simulink model "cpu1"  (R2022b)
settings: Solver=FixedStepDiscrete  StartTime=0.0  StopTime=Inf  RelTol=1e-3  EnableMultiTasking=on
model workspace (MAT data in the model file):
  x = 1
undefined symbols (not defined in the file): C28x, CPU1, CPU2, EALLOW, EDIS
libraries: c2837xDlib x11, dspstat3 x5, c280xlib x5, slpidlib x2, c2802xlib x2, svdutilitieslib x1, dspswit3 x1, idelinklib_common x1
(part 1 of 2)
settings Model: ExtModeTrigDuration=8  Creator=asus  LastModifiedBy=KH
settings SolverCC: AlgebraicLoopSolver=TrustRegion  AutoInsertRateTranBlk=on  InsertRTBMode=Always
settings OptimizationCC: DefaultUnderspecifiedDataType=single  EnhancedBackFolding=on  PassReuseOutputArgsAs=Individual arguments  MaxStackSize=1024  OptimizeBlockOrder=speed  DifferentSizesBufferReuse=on  OptimizationCustomize=off  DenormalBehavior=FlushToZero  EfficientTunableParamExpr=on
settings DebuggingCC: ParameterPrecisionLossMsg=none  ParameterTunabilityLossMsg=error  UnconnectedInputMsg=warning  UnconnectedOutputMsg=warning  UnconnectedLineMsg=warning  SFMachineParentedDataDiag=warning
settings HardwareCC: ProdBitPerChar=16  ProdBitPerInt=16  ProdBitPerPointer=32  ProdBitPerSizeT=32  ProdBitPerPtrDiffT=32  ProdLargestAtomicInteger=Integer  ProdLargestAtomicFloat=None  ProdWordSize=16  ProdLongLongMode=on  ProdHWDeviceType=Texas Instruments->C2000
settings ModelReferenceCC: EnableRefExpFcnMdlSchedulingChecks=on
settings SFSimCC: MATLABDynamicMemAlloc=off
settings RTWCC: Description=Embedded Coder  SystemTargetFile=ert.tlc  HardwareBoard=TI Delfino F28379D LaunchPad  TLCOptions=-aInlineSetEventsForThisBaseRateFcn=TLC_FALSE -aSuppressMultiTaskScheduler=TLC_FALSE -aRateBasedStepFcn=1  TemplateMakefile=ert_default_tmf  Toolchain=Texas Instruments Code Composer Studio (C2000)  DLArmComputeVersion=19.05
settings CodeAppCC: ForceParamTrailComments=on  IgnoreCustomStorageClasses=off  OperatorAnnotations=on  SimulinkDataObjDesc=on  SFDataObjDesc=on  InsertBlockDesc=on
settings ERTTargetCC: CodeReplacementLibrary=TI C28x  ExtModeTransport=3  ExtModeStaticAllocSize=10000

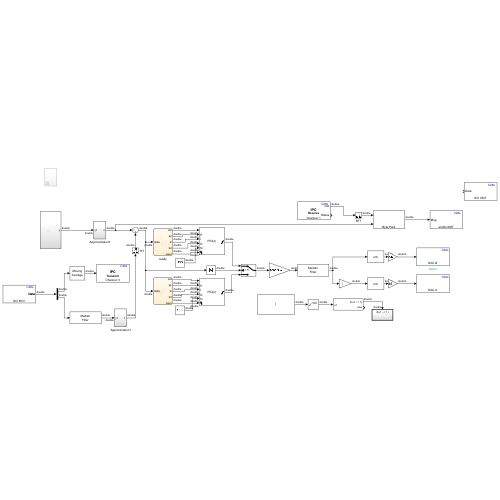
[thumbnail: Simulink's stored preview of the top-level diagram]
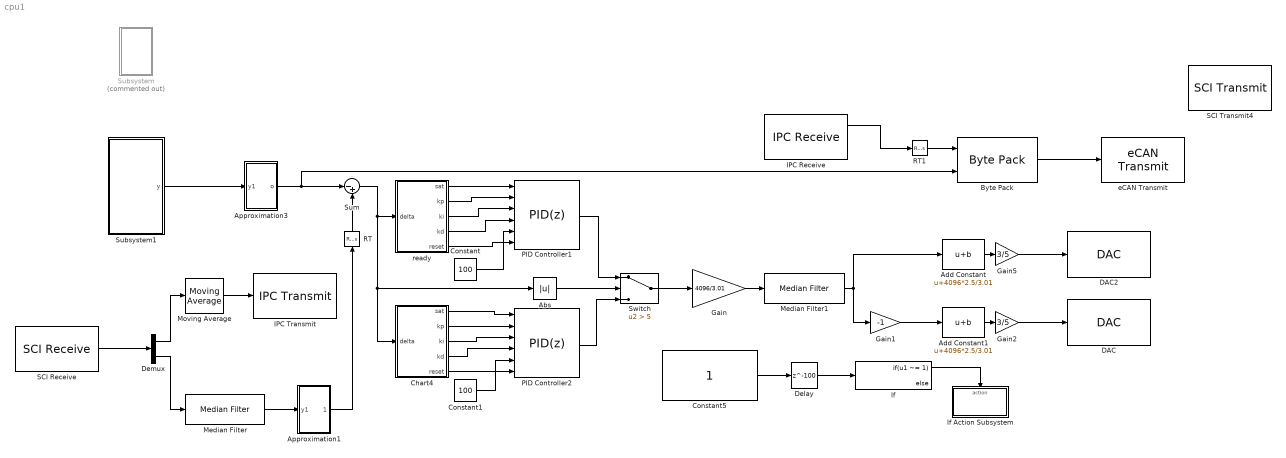
== system cpu1 ==
  " Approximation1" : Subsystem
  " Approximation3" : Subsystem
  Abs : Abs  SaturateOnIntegerOverflow=off
  Add Constant : Bias  Bias=4096*2.5/3.01  SaturateOnIntegerOverflow=off
  Add Constant1 : Bias  Bias=4096*2.5/3.01  SaturateOnIntegerOverflow=off
  Byte Pack : svdutilitieslib/Byte Pack  maskPackedDataType=uint16  datatypes={'single' 'single'}  byteAlign=4  blockPlatform=arduinoert
  Chart4 : Stateflow chart  TreatAsAtomicUnit=on
  Constant : Constant  Value=100
  Constant1 : Constant  Value=100
  Constant5 : Constant  OutDataTypeStr=Inherit: Inherit via back propagation
  DAC : c2837xDlib/DAC  channel=A  saturate=on
  DAC2 : c2837xDlib/DAC  channel=B  saturate=on
  Delay : Delay  DelayLength=100
  Demux : Demux  Outputs=2
  Gain : Gain  Gain=4096/3.01  OutDataTypeStr=single
  Gain1 : Gain  Gain=-1  OutDataTypeStr=single  SaturateOnIntegerOverflow=on
  Gain2 : Gain  Gain=3/5  OutDataTypeStr=single  SaturateOnIntegerOverflow=on
  Gain5 : Gain  Gain=3/5  OutDataTypeStr=single  SaturateOnIntegerOverflow=on
  IPC Receive : c2837xDlib/IPC Receive  blkParamProc=F2837x  SelectSource=C28x (CPU1/CPU2)  SelectChannel=1  DataType=single  DataLength=1  EnableBlocking=off  SampleTime=.001
  IPC Transmit : c2837xDlib/IPC Transmit  blkParamProc=F2837x  SelectDestination=C28x (CPU1/CPU2)  SelectChannel=0  EnableBlocking=off
  If : If  IfExpression=u1 ~= 1
  If Action Subsystem : Subsystem  TreatAsAtomicUnit=on
  Median Filter : dspstat3/Median Filter  WindowLength=3  SimulateUsing=Interpreted execution
  Median Filter1 : dspstat3/Median Filter  WindowLength=28  SimulateUsing=Interpreted execution
  Moving Average : dspstat3/Moving Average  Method=Sliding window  ForgettingFactorPort=off  SpecifyWindowLength=on  WindowLength=2  OverlapLength=1  AllowArbitraryInputLength=off  ForgettingFactor=0.9  SimulateUsing=Code generation
  PID Controller1 : slpidlib/PID Controller  Controller=PID  Form=Parallel  TimeDomain=Discrete-time  UseExternalTs=off  SampleTime=-1  IntegratorMethod=Forward Euler  FilterMethod=Forward Euler  ControllerParametersSource=external  P=0.0076  I=0.005  UseKiTs=off  D=0.00  N=100  UseFilter=on  TunerSelectOption=Transfer Function Based (PID Tuner App)  InitialConditionSource=internal  InitialConditionForIntegrator=0  InitialConditionForFilter=0  DifferentiatorICPrevScaledInput=0  ExternalReset=falling  TrackingMode=off  Kt=1  LimitOutput=on  SatLimitsSource=internal  UpperSaturationLimit=2.0  LowerSaturationLimit=-2.0  LinearizeAsGain=on  AntiWindupMode=clamping  Kb=1  LimitIntegrator=off  UpperIntegratorSaturationLimit=inf  LowerIntegratorSaturationLimit=-inf  PGainOutDataTypeStr=single  PProdOutDataTypeStr=single  POutMin=[]  POutMax=[]  IGainOutDataTypeStr=single  IProdOutDataTypeStr=single  IOutMin=[]  IOutMax=[]  DGainOutDataTypeStr=single  DProdOutDataTypeStr=single  DOutMin=[]  DOutMax=[]  NGainOutDataTypeStr=double  NProdOutDataTypeStr=double  NOutMin=[]  NOutMax=[]  SumOutDataTypeStr=single  SumOutMin=[]  SumOutMax=[]  SaturationOutDataTypeStr=single  SaturationOutMin=[]  SaturationOutMax=[]  PParamMin=[]  PParamMax=[]  IParamMin=[]  IParamMax=[]  DParamMin=[]  DParamMax=[]  NParamMin=[]  NParamMax=[]  KbParamMin=[]  KbParamMax=[]  KtParamMin=[]  KtParamMax=[]  KbOutMin=[]  KbOutMax=[]  KtOutMin=[]  KtOutMax=[]  IntegratorOutMin=[]  IntegratorOutMax=[]  FilterOutMin=[]  FilterOutMax=[]  SumI1OutMin=[]  SumI1OutMax=[]  SumI2OutMin=[]  SumI2OutMax=[]  SumI3OutMin=[]  SumI3OutMax=[]  SumI4OutMin=[]  SumI4OutMax=[]  SumDOutMin=[]  SumDOutMax=[]  DifferentiatorOutMin=[]  DifferentiatorOutMax=[]  FilterDiffOutCoefMin=[]  FilterDiffOutCoefMax=[]  ReciprocalOutMin=[]  ReciprocalOutMax=[]  SumDenOutMin=[]  SumDenOutMax=[]  SumNumOutMin=[]  SumNumOutMax=[]  DivideOutMin=[]  DivideOutMax=[]  UdiffTsProdOutMin=[]  UdiffTsProdOutMax=[]  NTsProdOutMin=[]  NTsProdOutMax=[]  UintegralTsProdOutMin=[]  UintegralTsProdOutMax=[]  UngainTsProdOutMin=[]  UngainTsProdOutMax=[]  ClampingZeroOutDataTypeStr=Inherit: Inherit via back propagation  ClampingZeroOutMin=[]  ClampingZeroOutMax=[]  FilterDenConstantOutDataTypeStr=Inherit: Inherit via back propagation  FilterDenConstantOutMin=[]  FilterDenConstantOutMax=[]  PCopyOutDataTypeStr=Inherit: Inherit via back propagation  PCopyOutMin=[]  PCopyOutMax=[]  NCopyOutDataTypeStr=Inherit: Inherit via back propagation  NCopyOutMin=[]  NCopyOutMax=[]  IntegratorContinuousStateAttributes=''  IntegratorStateMustResolveToSignalObject=off  IntegratorRTWStateStorageClass=Auto  FilterContinuousStateAttributes=''  FilterStateMustResolveToSignalObject=off  FilterRTWStateStorageClass=Auto  ParallelPVariant=ExternalParameters  IdealPVariant=Disabled  IVariant=ExternalParameters  DVariant=ExternalParameters  IntegratorVariant=Discrete  SatVariant=Enabled  AWVariant=DiscClampingParallel  PCopyVariant=Disabled  TRVariant=Disabled  FdbkBlocksVariant=Forward  IdealPFdbkVariant=Disabled  SatFdbkVariant=Disabled  DerivativeFilterVariant=ForwardEulerFilter  NVariant=ExternalParameters  NCopyVariant=Disabled  FilterICVariant=InternalICsFilter  IntegratorICVariant=InternalICs  ExternalResetVariant=ExternalReset  TRSumVariant=Passthrough  SumFdbkVariant=Disabled  SumVariant=Sum_PID  TsampFilterVariant=InternalTs  TsampNgainVariant=Passthrough  TsampIntegralVariant=Passthrough  ExternalSaturationOutDataTypeStr=Inherit: Same as second input
  PID Controller2 : slpidlib/PID Controller  Controller=PID  Form=Parallel  TimeDomain=Discrete-time  UseExternalTs=off  SampleTime=-1  IntegratorMethod=Forward Euler  FilterMethod=Forward Euler  ControllerParametersSource=external  P=0.0076  I=0.005  UseKiTs=off  D=0.00  N=100  UseFilter=on  TunerSelectOption=Transfer Function Based (PID Tuner App)  InitialConditionSource=internal  InitialConditionForIntegrator=0  InitialConditionForFilter=0  DifferentiatorICPrevScaledInput=0  ExternalReset=falling  TrackingMode=off  Kt=1  LimitOutput=on  SatLimitsSource=internal  UpperSaturationLimit=2.0  LowerSaturationLimit=-2.0  LinearizeAsGain=on  AntiWindupMode=none  Kb=1  LimitIntegrator=off  UpperIntegratorSaturationLimit=inf  LowerIntegratorSaturationLimit=-inf  PGainOutDataTypeStr=single  PProdOutDataTypeStr=single  POutMin=[]  POutMax=[]  IGainOutDataTypeStr=single  IProdOutDataTypeStr=single  IOutMin=[]  IOutMax=[]  DGainOutDataTypeStr=single  DProdOutDataTypeStr=single  DOutMin=[]  DOutMax=[]  NGainOutDataTypeStr=double  NProdOutDataTypeStr=double  NOutMin=[]  NOutMax=[]  SumOutDataTypeStr=single  SumOutMin=[]  SumOutMax=[]  SaturationOutDataTypeStr=single  SaturationOutMin=[]  SaturationOutMax=[]  PParamMin=[]  PParamMax=[]  IParamMin=[]  IParamMax=[]  DParamMin=[]  DParamMax=[]  NParamMin=[]  NParamMax=[]  KbParamMin=[]  KbParamMax=[]  KtParamMin=[]  KtParamMax=[]  KbOutMin=[]  KbOutMax=[]  KtOutMin=[]  KtOutMax=[]  IntegratorOutMin=[]  IntegratorOutMax=[]  FilterOutMin=[]  FilterOutMax=[]  SumI1OutMin=[]  SumI1OutMax=[]  SumI2OutMin=[]  SumI2OutMax=[]  SumI3OutMin=[]  SumI3OutMax=[]  SumI4OutMin=[]  SumI4OutMax=[]  SumDOutMin=[]  SumDOutMax=[]  DifferentiatorOutMin=[]  DifferentiatorOutMax=[]  FilterDiffOutCoefMin=[]  FilterDiffOutCoefMax=[]  ReciprocalOutMin=[]  ReciprocalOutMax=[]  SumDenOutMin=[]  SumDenOutMax=[]  SumNumOutMin=[]  SumNumOutMax=[]  DivideOutMin=[]  DivideOutMax=[]  UdiffTsProdOutMin=[]  UdiffTsProdOutMax=[]  NTsProdOutMin=[]  NTsProdOutMax=[]  UintegralTsProdOutMin=[]  UintegralTsProdOutMax=[]  UngainTsProdOutMin=[]  UngainTsProdOutMax=[]  ClampingZeroOutDataTypeStr=Inherit: Inherit via back propagation  ClampingZeroOutMin=[]  ClampingZeroOutMax=[]  FilterDenConstantOutDataTypeStr=Inherit: Inherit via back propagation  FilterDenConstantOutMin=[]  FilterDenConstantOutMax=[]  PCopyOutDataTypeStr=Inherit: Inherit via back propagation  PCopyOutMin=[]  PCopyOutMax=[]  NCopyOutDataTypeStr=Inherit: Inherit via back propagation  NCopyOutMin=[]  NCopyOutMax=[]  IntegratorContinuousStateAttributes=''  IntegratorStateMustResolveToSignalObject=off  IntegratorRTWStateStorageClass=Auto  FilterContinuousStateAttributes=''  FilterStateMustResolveToSignalObject=off  FilterRTWStateStorageClass=Auto  ParallelPVariant=ExternalParameters  IdealPVariant=Disabled  IVariant=ExternalParameters  DVariant=ExternalParameters  IntegratorVariant=Discrete  SatVariant=Enabled  AWVariant=Passthrough  PCopyVariant=Disabled  TRVariant=Disabled  FdbkBlocksVariant=Forward  IdealPFdbkVariant=Disabled  SatFdbkVariant=Disabled  DerivativeFilterVariant=ForwardEulerFilter  NVariant=ExternalParameters  NCopyVariant=Disabled  FilterICVariant=InternalICsFilter  IntegratorICVariant=InternalICs  ExternalResetVariant=ExternalReset  TRSumVariant=Passthrough  SumFdbkVariant=Disabled  SumVariant=Sum_PID  TsampFilterVariant=InternalTs  TsampNgainVariant=Passthrough  TsampIntegralVariant=Passthrough  ExternalSaturationOutDataTypeStr=Inherit: Same as second input
  RT : RateTransition  OutPortSampleTime=0.001
  RT1 : RateTransition  OutPortSampleTime=0.001
  SCI Receive : c280xlib/SCI Receive  sciModule=A  dataHead=''  headerCheckMaxCount=16  dataTail=''  dataType=single  dataLenOptions=Length via dialog  dataDim=2  maxDataLength=1  initValue=0  errOption=Output the last received value  errValue=0  sampleTime=0.1  blockingMode=on  timeOut=inf  outputStatus=off
  SCI Transmit4 : c280xlib/SCI Transmit  sciModule=A  dataHead=''  dataTail=''  blockingMode=on  outputStatus=off
  Subsystem : Subsystem  Commented=on
  Subsystem1 : Subsystem
  Sum : Sum  Inputs=|-+
  Switch : Switch  Criteria=u2 > Threshold  Threshold=5  SaturateOnIntegerOverflow=off  InputSameDT=off
  eCAN Transmit : c280xlib/eCAN Transmit  chipFamily=C280x  useModule=eCAN_A  mailboxNo=1  messageID=bin2dec('111000111')  messageType=Standard (11-bit identifier)  enableBlockingMode=off  postInterrupt=off  interruptLine=0
      settings: LibrarySourceBlock=c2837xDlib/eCAN Transmit
  ready : Stateflow chart  TreatAsAtomicUnit=on
  wires:
  If/1 -> If Action Subsystem/Action
  Delay/1 -> If/1
  Constant5/1 -> Delay/1
  Add Constant1/1 -> Gain2/1
  Add Constant/1 -> Gain5/1
  Gain1/1 -> Add Constant1/1
  Gain5/1 -> DAC2/1
  Gain2/1 -> DAC/1
  Constant/1 -> PID Controller1/5
  PID Controller1/1 -> Switch/1
  ready/2(kp) -> PID Controller1/2
  ready/3(ki) -> PID Controller1/3
  ready/4(kd) -> PID Controller1/4
  ready/1(sat) -> PID Controller1/1
  ready/5(reset) -> PID Controller1/6
  " Approximation1"/1(Out1) -> RT/1
  RT/1 -> Sum/2
  Subsystem1/1(y) -> " Approximation3"/1(y1)
  Median Filter/1 -> " Approximation1"/1(y1)
  Gain/1 -> Median Filter1/1
  " Approximation3"/1(o) -> Byte Pack/2, Sum/1
  Switch/1 -> Gain/1
  Chart4/5(reset) -> PID Controller2/6
  Chart4/1(sat) -> PID Controller2/1
  Chart4/3(ki) -> PID Controller2/3
  Constant1/1 -> PID Controller2/5
  Chart4/4(kd) -> PID Controller2/4
  Sum/1 -> Chart4/1(delta), Abs/1, ready/1(delta)
  Chart4/2(kp) -> PID Controller2/2
  PID Controller2/1 -> Switch/3
  Abs/1 -> Switch/2
  Median Filter1/1 -> Gain1/1, Add Constant/1
  Demux/1 -> Moving Average/1
  Moving Average/1 -> IPC Transmit/1
  IPC Receive/1 -> RT1/1
  RT1/1 -> Byte Pack/1
  SCI Receive/1 -> Demux/1
  Demux/2 -> Median Filter/1
  Byte Pack/1 -> eCAN Transmit/1

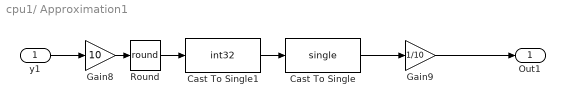
== system cpu1/ Approximation1 ==
  y1 : Inport
  Cast To Single : DataTypeConversion  OutDataTypeStr=single  SaturateOnIntegerOverflow=off  RndMeth=Floor
  Cast To Single1 : DataTypeConversion  OutDataTypeStr=int32  SaturateOnIntegerOverflow=off  RndMeth=Floor
  Gain8 : Gain  Gain=10
  Gain9 : Gain  Gain=1/10
  Round : Rounding  Operator=round
  Out1 : Outport
  wires:
  y1/1 -> Gain8/1
  Gain8/1 -> Round/1
  Round/1 -> Cast To Single1/1
  Cast To Single1/1 -> Cast To Single/1
  Cast To Single/1 -> Gain9/1
  Gain9/1 -> Out1/1

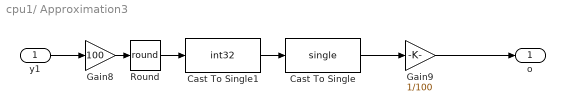
== system cpu1/ Approximation3 ==
  y1 : Inport
  Cast To Single : DataTypeConversion  OutDataTypeStr=single  SaturateOnIntegerOverflow=off  RndMeth=Floor
  Cast To Single1 : DataTypeConversion  OutDataTypeStr=int32  SaturateOnIntegerOverflow=off  RndMeth=Floor
  Gain8 : Gain  Gain=100
  Gain9 : Gain  Gain=1/100
  Round : Rounding  Operator=round
  o : Outport
  wires:
  Gain9/1 -> o/1
  Cast To Single/1 -> Gain9/1
  Cast To Single1/1 -> Cast To Single/1
  Round/1 -> Cast To Single1/1
  Gain8/1 -> Round/1
  y1/1 -> Gain8/1

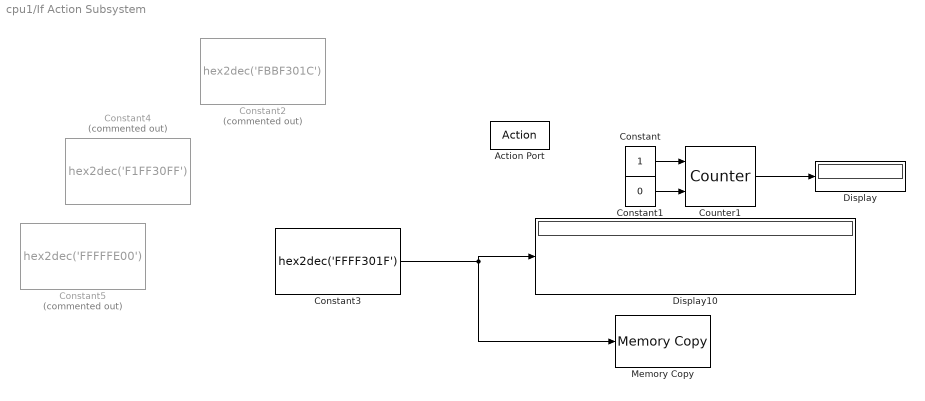
== system cpu1/If Action Subsystem ==
  Action Port : ActionPort  ActionPortLabel=if(u1 ~= 1)
  Constant : Constant
  Constant1 : Constant  Value=0
  Constant2 : Constant  Commented=on  Value=hex2dec('FBBF301C')  OutDataTypeStr=uint32
  Constant3 : Constant  Value=hex2dec('FFFF301F')  OutDataTypeStr=uint32
  Constant4 : Constant  Commented=on  Value=hex2dec('F1FF30FF')  OutDataTypeStr=uint32
  Constant5 : Constant  Commented=on  Value=hex2dec('FFFFFE00')  OutDataTypeStr=uint32
  Counter1 : dspswit3/Counter  Direction=Up  CountEvent=Rising edge  CounterSize=User defined  MaxCount=255  InitialCount=0  Output=Count  HitValue=32  ResetInput=on  SamplesPerFrame=1  Ts=1  CntDtype=double  HitDtype=Logical
  Display : Display
  Display10 : Display
      settings: Format=binary (Stored Integer)
  Memory Copy : idelinklib_common/Memory Copy  copyFrom=Input port  copyFromAddressSource=Specify via dialog  copyFromAddress=hex2dec('00001000')  copyFromSrcCode=myVariableSrc  dataTypeFrom=uint32  dataDimensionFrom=1  useOffsetFrom=off  offsetFromSrc=Specify via dialog  offsetFrom=0  strideFrom=1  copyTo=Specified address  copyToAddressSource=Specify via dialog  copyToAddress=hex2dec('00007C0C')  copyToSrcCode=myVariableDst  dataTypeTo=uint32  useOffsetTo=off  offsetToSrc=Specify via dialog  offsetTo=0  strideTo=1  sampleTime=inf  useInitValue=off  initValueSrc=Specify constant value  initValue=1  initValueSrcCode=myInitValueVariable  useAsMask=off  maskOperator=bitwise AND  useTermValue=off  termValue=1  isRealtimeEnabled=off  emitCCBeforeWrite=on  CCBeforeWrite=EALLOW;  emitCCAfterWrite=on  CCAfterWrite=EDIS;
  wires:
  Constant3/1 -> Display10/1, Memory Copy/1
  Constant1/1 -> Counter1/2
  Constant/1 -> Counter1/1
  Counter1/1 -> Display/1

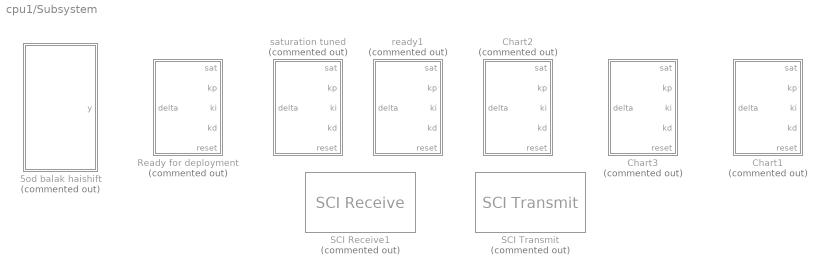
== system cpu1/Subsystem ==
  5od balak haishift : Subsystem  Commented=on
  Chart1 : Stateflow chart  Commented=on  TreatAsAtomicUnit=on
  Chart2 : Stateflow chart  Commented=on  TreatAsAtomicUnit=on
  Chart3 : Stateflow chart  Commented=on  TreatAsAtomicUnit=on
  Ready for deployment : Stateflow chart  Commented=on  TreatAsAtomicUnit=on
  SCI Receive1 : c280xlib/SCI Receive  Commented=on  sciModule=B  dataHead=''  dataTail=''  dataType=single  dataDim=1  initValue=0  errOption=Output the last received value  errValue=0  sampleTime=0.1  outputStatus=off  postInterrupt=off  numFifo=1
  SCI Transmit : c280xlib/SCI Transmit  Commented=on  sciModule=B  dataHead=''  dataTail=''  postInterrupt=off  numFifo=1
  ready1 : Stateflow chart  Commented=on  TreatAsAtomicUnit=on
  saturation tuned : Stateflow chart  Commented=on  TreatAsAtomicUnit=on

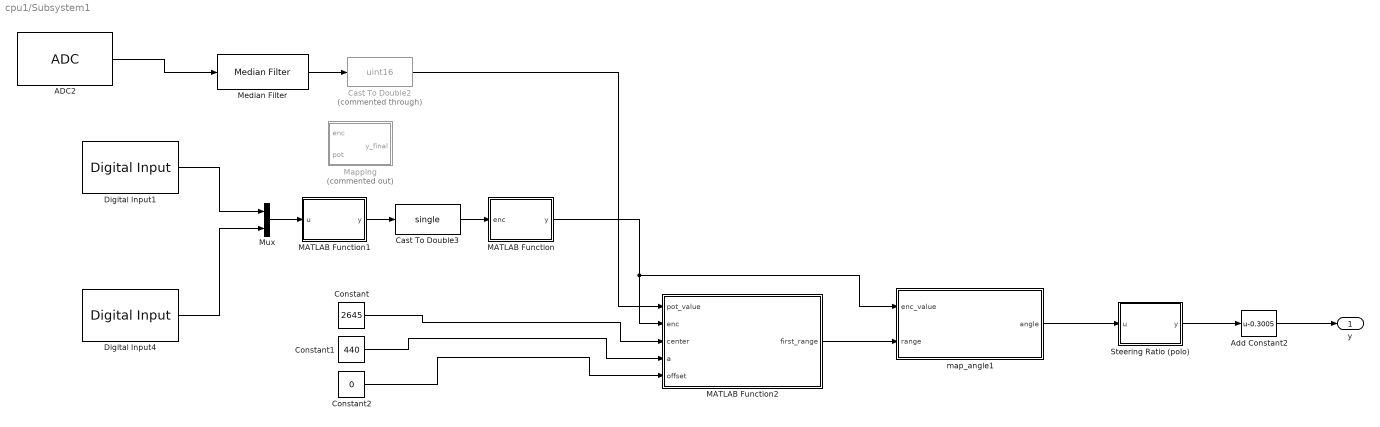
== system cpu1/Subsystem1 ==
  ADC2 : c2802xlib/ADC  blkParamProc=C2000_Type4  ADCModule=A  samplingMode=Single sample mode  ADCResolution=12-bit (Single-ended input)  useSOC1=SOC0  useSOC2=SOC0_SOC1  SOCAcquisitionWindow=15  SOCTriggerSource=Software  SOCInterruptTrigger=No ADCINT  Ts=0.001  dType=single  postInterrupt=off  interruptSel=ADCINT1  ADCINTContinuous=on  endma=off  chdma=1  conv1=ADCINA0  conv2=ADCINA0 and ADCINB0  conv1_Type4=ADCIN2  conv2_Type4=ADCIN0 and ADCIN1
  Add Constant2 : Bias  Bias=-0.3005  SaturateOnIntegerOverflow=off
  Cast To Double2 : DataTypeConversion  Commented=through  OutDataTypeStr=uint16  SaturateOnIntegerOverflow=off  RndMeth=Floor
  Cast To Double3 : DataTypeConversion  OutDataTypeStr=single  SaturateOnIntegerOverflow=off  RndMeth=Floor
  Constant : Constant  Value=2645  OutDataTypeStr=single
  Constant1 : Constant  Value=440  OutDataTypeStr=single
  Constant2 : Constant  Value=0  OutDataTypeStr=single
  Digital Input1 : c2837xDlib/Digital Input  GPIO_Number=GPIO0~GPIO7  GPIO_Bit0=off  GPIO_Bit1=off  GPIO_Bit2=off  GPIO_Bit3=off  GPIO_Bit4=off  GPIO_Bit5=on  GPIO_Bit6=on  GPIO_Bit7=on  sampleTime=0.001  dataType=int32  GPIO_Bit0_Qualification=Sync to SYSCLKOUT  GPIO_Bit1_Qualification=Sync to SYSCLKOUT  GPIO_Bit2_Qualification=Sync to SYSCLKOUT  GPIO_Bit3_Qualification=Sync to SYSCLKOUT  GPIO_Bit4_Qualification=Sync to SYSCLKOUT  GPIO_Bit5_Qualification=Sync to SYSCLKOUT  GPIO_Bit6_Qualification=Sync to SYSCLKOUT  GPIO_Bit7_Qualification=Sync to SYSCLKOUT  Qualification_Period=-1
  Digital Input4 : c2837xDlib/Digital Input  GPIO_Number=GPIO8~GPIO15  GPIO_Bit0=on  GPIO_Bit1=on  GPIO_Bit2=on  GPIO_Bit3=on  GPIO_Bit4=off  GPIO_Bit5=off  GPIO_Bit6=on  GPIO_Bit7=on  sampleTime=0.001  dataType=int32  GPIO_Bit0_Qualification=Sync to SYSCLKOUT  GPIO_Bit1_Qualification=Sync to SYSCLKOUT  GPIO_Bit2_Qualification=Sync to SYSCLKOUT  GPIO_Bit3_Qualification=Sync to SYSCLKOUT  GPIO_Bit4_Qualification=Sync to SYSCLKOUT  GPIO_Bit5_Qualification=Sync to SYSCLKOUT  GPIO_Bit6_Qualification=Sync to SYSCLKOUT  GPIO_Bit7_Qualification=Sync to SYSCLKOUT  Qualification_Period=-1
  MATLAB Function : MATLAB Function  TreatAsAtomicUnit=on
  MATLAB Function1 : MATLAB Function  TreatAsAtomicUnit=on
  MATLAB Function2 : MATLAB Function  TreatAsAtomicUnit=on
  Mapping : MATLAB Function  Commented=on  TreatAsAtomicUnit=on
  Median Filter : dspstat3/Median Filter  WindowLength=5  SimulateUsing=Interpreted execution
  Mux : Mux  Inputs=2
  Steering Ratio (polo) : MATLAB Function  TreatAsAtomicUnit=on
  map_angle1 : MATLAB Function  TreatAsAtomicUnit=on
  y : Outport
  wires:
  ADC2/1 -> Median Filter/1
  Digital Input4/1 -> Mux/2
  Median Filter/1 -> Cast To Double2/1
  Digital Input1/1 -> Mux/1
  Mux/1 -> MATLAB Function1/1(u)
  Steering Ratio (polo)/1(y) -> Add Constant2/1
  MATLAB Function1/1(y) -> Cast To Double3/1
  Cast To Double2/1 -> MATLAB Function2/1(pot_value)
  Cast To Double3/1 -> MATLAB Function/1(enc)
  Add Constant2/1 -> y/1
  MATLAB Function/1(y) -> MATLAB Function2/2(enc), map_angle1/1(enc_value)
  map_angle1/1(angle) -> Steering Ratio (polo)/1(u)
  Constant/1 -> MATLAB Function2/3(center)
  Constant1/1 -> MATLAB Function2/4(a)
  Constant2/1 -> MATLAB Function2/5(offset)
  MATLAB Function2/1(first_range) -> map_angle1/2(range)

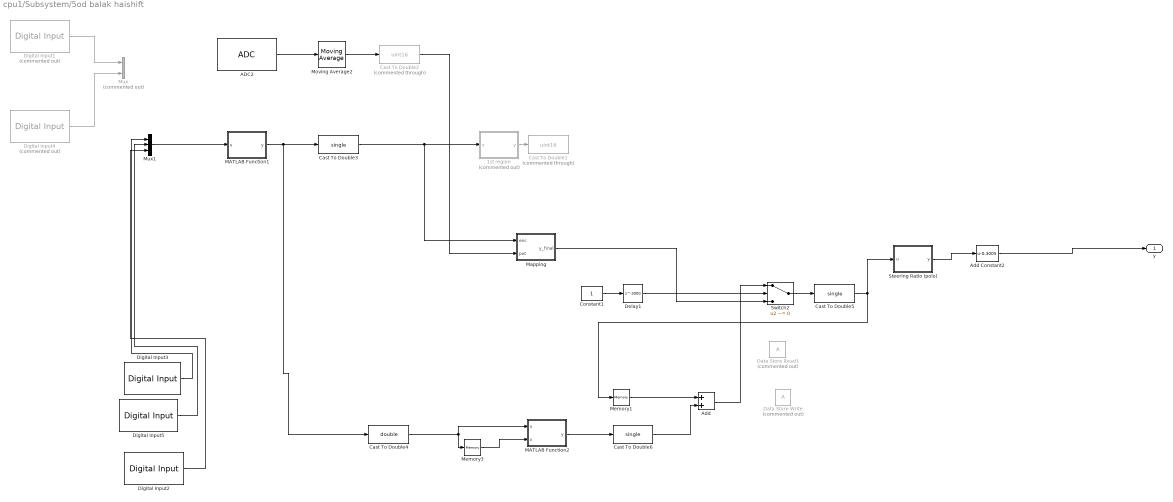
== system cpu1/Subsystem/5od balak haishift ==
  1st region : MATLAB Function  Commented=on  TreatAsAtomicUnit=on
  ADC2 : c2802xlib/ADC  blkParamProc=C2000_Type4  ADCModule=A  samplingMode=Single sample mode  ADCResolution=12-bit (Single-ended input)  useSOC1=SOC0  useSOC2=SOC0_SOC1  SOCAcquisitionWindow=15  SOCTriggerSource=Software  SOCInterruptTrigger=No ADCINT  Ts=0.001  dType=single  postInterrupt=off  interruptSel=ADCINT1  ADCINTContinuous=on  endma=off  chdma=1  conv1=ADCINA0  conv2=ADCINA0 and ADCINB0  conv1_Type4=ADCIN2  conv2_Type4=ADCIN0 and ADCIN1
  Add : Sum
  Add Constant2 : Bias  Bias=-0.3005  SaturateOnIntegerOverflow=off
  Cast To Double1 : DataTypeConversion  Commented=through  OutDataTypeStr=uint16  SaturateOnIntegerOverflow=off  RndMeth=Floor
  Cast To Double2 : DataTypeConversion  Commented=through  OutDataTypeStr=uint16  SaturateOnIntegerOverflow=off  RndMeth=Floor
  Cast To Double3 : DataTypeConversion  OutDataTypeStr=single  SaturateOnIntegerOverflow=off  RndMeth=Floor
  Cast To Double4 : DataTypeConversion  OutDataTypeStr=double  SaturateOnIntegerOverflow=off  RndMeth=Floor
  Cast To Double5 : DataTypeConversion  OutDataTypeStr=single  SaturateOnIntegerOverflow=off  RndMeth=Floor
  Cast To Double6 : DataTypeConversion  OutDataTypeStr=single  SaturateOnIntegerOverflow=off  RndMeth=Floor
  Constant1 : Constant  OutDataTypeStr=Inherit: Inherit via back propagation
  Data Store Read1 : DataStoreRead  Commented=on  DataStoreElements=A  IndexOptions=Index vector (dialog)  Indices=1  OutputSizes=1
  Data Store Write : DataStoreWrite  Commented=on  DataStoreElements=A  IndexOptions=Index vector (dialog)  Indices=1  OutputSizes=1
  Delay1 : Delay  DelayLength=3000
  Digital Input1 : c2837xDlib/Digital Input  Commented=on  GPIO_Number=GPIO0~GPIO7  GPIO_Bit0=off  GPIO_Bit1=off  GPIO_Bit2=off  GPIO_Bit3=off  GPIO_Bit4=off  GPIO_Bit5=on  GPIO_Bit6=on  GPIO_Bit7=on  sampleTime=0.001  dataType=int32  GPIO_Bit0_Qualification=Sync to SYSCLKOUT  GPIO_Bit1_Qualification=Sync to SYSCLKOUT  GPIO_Bit2_Qualification=Sync to SYSCLKOUT  GPIO_Bit3_Qualification=Sync to SYSCLKOUT  GPIO_Bit4_Qualification=Sync to SYSCLKOUT  GPIO_Bit5_Qualification=Sync to SYSCLKOUT  GPIO_Bit6_Qualification=Sync to SYSCLKOUT  GPIO_Bit7_Qualification=Sync to SYSCLKOUT  Qualification_Period=-1
  Digital Input2 : c2837xDlib/Digital Input  GPIO_Number=GPIO24~GPIO31  GPIO_Bit0=off  GPIO_Bit1=on  GPIO_Bit2=off  GPIO_Bit3=off  GPIO_Bit4=off  GPIO_Bit5=off  GPIO_Bit6=off  GPIO_Bit7=off  sampleTime=0.001  dataType=int32  GPIO_Bit0_Qualification=Sync to SYSCLKOUT  GPIO_Bit1_Qualification=Sync to SYSCLKOUT  GPIO_Bit2_Qualification=Sync to SYSCLKOUT  GPIO_Bit3_Qualification=Sync to SYSCLKOUT  GPIO_Bit4_Qualification=Sync to SYSCLKOUT  GPIO_Bit5_Qualification=Sync to SYSCLKOUT  GPIO_Bit6_Qualification=Sync to SYSCLKOUT  GPIO_Bit7_Qualification=Sync to SYSCLKOUT  Qualification_Period=-1
  Digital Input3 : c2837xDlib/Digital Input  GPIO_Number=GPIO8~GPIO15  GPIO_Bit0=on  GPIO_Bit1=on  GPIO_Bit2=on  GPIO_Bit3=on  GPIO_Bit4=off  GPIO_Bit5=off  GPIO_Bit6=on  GPIO_Bit7=on  sampleTime=0.001  dataType=int32  GPIO_Bit0_Qualification=Sync to SYSCLKOUT  GPIO_Bit1_Qualification=Sync to SYSCLKOUT  GPIO_Bit2_Qualification=Sync to SYSCLKOUT  GPIO_Bit3_Qualification=Sync to SYSCLKOUT  GPIO_Bit4_Qualification=Sync to SYSCLKOUT  GPIO_Bit5_Qualification=Sync to SYSCLKOUT  GPIO_Bit6_Qualification=Sync to SYSCLKOUT  GPIO_Bit7_Qualification=Sync to SYSCLKOUT  Qualification_Period=-1
  Digital Input4 : c2837xDlib/Digital Input  Commented=on  GPIO_Number=GPIO8~GPIO15  GPIO_Bit0=on  GPIO_Bit1=on  GPIO_Bit2=on  GPIO_Bit3=on  GPIO_Bit4=off  GPIO_Bit5=off  GPIO_Bit6=on  GPIO_Bit7=on  sampleTime=0.001  dataType=int32  GPIO_Bit0_Qualification=Sync to SYSCLKOUT  GPIO_Bit1_Qualification=Sync to SYSCLKOUT  GPIO_Bit2_Qualification=Sync to SYSCLKOUT  GPIO_Bit3_Qualification=Sync to SYSCLKOUT  GPIO_Bit4_Qualification=Sync to SYSCLKOUT  GPIO_Bit5_Qualification=Sync to SYSCLKOUT  GPIO_Bit6_Qualification=Sync to SYSCLKOUT  GPIO_Bit7_Qualification=Sync to SYSCLKOUT  Qualification_Period=-1
  Digital Input5 : c2837xDlib/Digital Input  GPIO_Number=GPIO24~GPIO31  GPIO_Bit0=off  GPIO_Bit1=off  GPIO_Bit2=on  GPIO_Bit3=on  GPIO_Bit4=off  GPIO_Bit5=off  GPIO_Bit6=off  GPIO_Bit7=off  sampleTime=0.001  dataType=int32  GPIO_Bit0_Qualification=Sync to SYSCLKOUT  GPIO_Bit1_Qualification=Sync to SYSCLKOUT  GPIO_Bit2_Qualification=Sync to SYSCLKOUT  GPIO_Bit3_Qualification=Sync to SYSCLKOUT  GPIO_Bit4_Qualification=Sync to SYSCLKOUT  GPIO_Bit5_Qualification=Sync to SYSCLKOUT  GPIO_Bit6_Qualification=Sync to SYSCLKOUT  GPIO_Bit7_Qualification=Sync to SYSCLKOUT  Qualification_Period=-1
  MATLAB Function1 : MATLAB Function  TreatAsAtomicUnit=on
  MATLAB Function2 : MATLAB Function  TreatAsAtomicUnit=on
  Mapping : MATLAB Function  TreatAsAtomicUnit=on
  Memory1 : Memory  InheritSampleTime=on
  Memory3 : Memory  InheritSampleTime=on
  Moving Average2 : dspstat3/Moving Average  Method=Sliding window  ForgettingFactorPort=off  SpecifyWindowLength=on  WindowLength=250  ForgettingFactor=0.9  SimulateUsing=Code generation
  Mux : Mux  Commented=on  Inputs=2
  Mux1 : Mux  Inputs=3
  Steering Ratio (polo) : MATLAB Function  TreatAsAtomicUnit=on
  Switch2 : Switch  Criteria=u2 ~= 0  SaturateOnIntegerOverflow=off  InputSameDT=off
  y : Outport
  wires:
  Add Constant2/1 -> y/1
  Cast To Double3/1 -> 1st region/1(x), Mapping/1(enc)
  Cast To Double2/1 -> Mapping/2(pot)
  Cast To Double6/1 -> Add/2
  Cast To Double4/1 -> MATLAB Function2/1(u), Memory3/1
  MATLAB Function2/1(y) -> Cast To Double6/1
  Memory3/1 -> MATLAB Function2/2(x)
  Digital Input5/1 -> Mux1/2
  Digital Input3/1 -> Mux1/1
  Digital Input2/1 -> Mux1/3
  Add/1 -> Switch2/1
  Memory1/1 -> Add/1
  Mapping/1(y_final) -> Switch2/3
  Cast To Double5/1 -> Steering Ratio (polo)/1(u), Memory1/1
  Delay1/1 -> Switch2/2
  Constant1/1 -> Delay1/1
  Switch2/1 -> Cast To Double5/1
  MATLAB Function1/1(y) -> Cast To Double4/1, Cast To Double3/1
  Steering Ratio (polo)/1(y) -> Add Constant2/1
  1st region/1(y) -> Cast To Double1/1
  Mux1/1 -> MATLAB Function1/1(u)
  Digital Input1/1 -> Mux/1
  Moving Average2/1 -> Cast To Double2/1
  Digital Input4/1 -> Mux/2
  ADC2/1 -> Moving Average2/1

== stateflow chart cpu1/Subsystem/Chart1 ==
  state init
    f20 = 0;
    f15 = 0;
    f10 = 0;
    kp = 0;
    ki = 0;
    kd = 0;
    sat = 0;
  state state10
    if delta > 0
    sat = 5;
    else
    sat = -5;
    end
    if f20 == 1 && f15==1 && f10==1
    kp = 0.07;
    elseif f20==0 && f15==1 && f10==1
    kp = 0.08;
    elseif f20==0 && f15==0 && f10==1
    kp = 0.08;
    else
    kp= 0.09;
    end
    reset =0;
  state state13
    sat = double(delta);
    kp= 0.35;
    if (abs(delta)<=0.5)
    ki=0.15;
    else
    ki=0.10;
    end
    reset = 1;
  state state12
    if delta > 0
    sat = 1;
    else
    sat = -1;
    end
    kp= 0.3;
    reset =0;
  state state9
    if delta > 0
    sat = 15;
    else
    sat = -15;
    end
    if f20 == 1
    kp = 0.03;
    else
    kp = 0.04;
    end
    f15 = 1;
    reset=0;
  state state11
    if delta > 0
    sat = 2;
    else
    sat = -2;
    end
    if f20 == 1 && f15==1 && f10==1
    kp = 0.15;
    elseif f20==0 && f15==1 && f10==1
    kp = 0.2;
    elseif f20==0 && f15==0 && f10==1
    kp = 0.2;
    else
    kp= 0.22;
    end
    reset =0;
  state state8
    if delta > 0
    sat = 10;
    else
    sat = -10;
    end
    if f20 == 1 && f15==1
    kp = 0.04;
    elseif f15==1 && f20==0
    kp = 0.045;
    else
    kp = 0.05;
    end
    f10 = 1;
    reset=0;
  state else
    kp=0;
    sat=0;
    reset =1;
  state state1
    if delta > 0
    sat = 20;
    else
    sat = -20;
    end
    kp = 0.025;
    f20 = 1;
    reset=0;
  (default) -> init
  init -> (junction 7)
  (junction 7) -> state10 [order 7] : [abs(delta)>=5 && abs(delta)<10]
  (junction 7) -> state12 [order 4] : [abs(delta)>=1 && abs(delta)<2]
  (junction 7) -> state11 [order 5] : [abs(delta)>=2 && abs(delta)<5]
  (junction 7) -> state9 [order 3] : [abs(delta)<20 && abs(delta)>=15]
  (junction 7) -> state8 [order 2] : [abs(delta)>=10 && abs(delta)<15]
  (junction 7) -> state1 [order 1] : [abs(delta)>=20]
  (junction 7) -> state13 [order 6] : [abs(delta)>=0.04 && abs(delta)<1]
  else -> (junction 7) : [~(abs(delta)<0.04)]{f20=0,f15=0,f10=0,reset=0}
  state12 -> state10 [order 4] : [abs(delta)>=5 && abs(delta)<10]
  state12 -> state13 [order 6] : [abs(delta)>=0.04 && abs(delta)<1]
  state13 -> state10 [order 6] : [abs(delta)>=5 && abs(delta)<10]{f20=0,f15=0,f10=0,ki=0}
  state10 -> state12 [order 6] : [abs(delta)>=1 && abs(delta)<2]
  state11 -> state13 [order 7] : [abs(delta)>=0.04 && abs(delta)<1]
  state12 -> state1 [order 5] : [abs(delta)>=20]
  state8 -> state10 [order 3] : [abs(delta)>=5 && abs(delta)<10]
  state8 -> state13 [order 7] : [abs(delta)>=0.04 && abs(delta)<1]
  state1 -> state12 [order 2] : [abs(delta)>=1 && abs(delta)<2]
  state11 -> state10 [order 2] : [abs(delta)>=5 && abs(delta)<10]{f20=0,f15=0,f10=0}
  state10 -> state1 [order 3] : [abs(delta)>=20]{f20=0,f15=0,f10=0}
  state10 -> state9 [order 2] : [abs(delta)<20 && abs(delta)>=15]{f20=0,f15=0,f10=0}
  state10 -> state8 [order 1] : [abs(delta)>=10 && abs(delta)<15]{f20=0,f15=0,f10=0}
  state10 -> state11 [order 5] : [abs(delta)>=2 && abs(delta)<5]
  state9 -> state12 [order 4] : [abs(delta)>=1 && abs(delta)<2]
  state13 -> state12 [order 1] : [abs(delta)>=1 && abs(delta)<2]{f20=0,f15=0,f10=0,ki=0}
  state13 -> state9 [order 2] : [abs(delta)<20 && abs(delta)>=15]{f20=0,f15=0,f10=0,ki=0}
  state12 -> else [order 7] : [abs(delta)<0.04]
  state9 -> state10 [order 6] : [abs(delta)>=5 && abs(delta)<10]{f20=0,f15=0,f10=0}
  state9 -> state13 [order 2] : [abs(delta)>=0.04 && abs(delta)<1]
  state8 -> state12 [order 6] : [abs(delta)>=1 && abs(delta)<2]
  state13 -> state8 [order 5] : [abs(delta)>=10 && abs(delta)<15]{f20=0,f15=0,f10=0,ki=0}
  state10 -> else [order 4] : [abs(delta)<0.04]
  state13 -> state11 [order 3] : [abs(delta)>=2 && abs(delta)<5]{f20=0,f15=0,f10=0,ki=0}
  state1 -> state10 [order 5] : [abs(delta)>=5 && abs(delta)<10]{f20=0}
  state10 -> state13 [order 7] : [abs(delta)>=0.04 && abs(delta)<1]
  state11 -> state12 [order 6] : [abs(delta)>=1 && abs(delta)<2]
  state13 -> state1 [order 4] : [abs(delta)>=20]{f20=0,f15=0,f10=0,ki=0}
  state13 -> else [order 7] : [abs(delta)<0.04]{ki=0}
  state12 -> state9 [order 1] : [abs(delta)<20 && abs(delta)>=15]
  state12 -> state8 [order 3] : [abs(delta)>=10 && abs(delta)<15]
  state12 -> state11 [order 2] : [abs(delta)>=2 && abs(delta)<5]
  state1 -> state8 [order 4] : [abs(delta)>=10 && abs(delta)<15]{f20=0}
  state8 -> state9 [order 2] : [abs(delta)<20 && abs(delta)>=15]{f20=0}
  state11 -> else [order 1] : [abs(delta)<0.04]
  state9 -> state8 [order 1] : [abs(delta)>=10 && abs(delta)<15]
  state9 -> else [order 7] : [abs(delta)<0.04]
  state8 -> else [order 5] : [abs(delta)<0.04]
  state1 -> else [order 6] : [abs(delta)<0.04]
  state11 -> state9 [order 4] : [abs(delta)<20 && abs(delta)>=15]{f20=0,f15=0,f10=0}
  state1 -> state9 [order 1] : [abs(delta)<20 && abs(delta)>=15]
  state9 -> state1 [order 3] : [abs(delta)>=20]
  state9 -> state11 [order 5] : [abs(delta)>=2 && abs(delta)<5]
  state8 -> state11 [order 4] : [abs(delta)>=2 && abs(delta)<5]
  state8 -> state1 [order 1] : [abs(delta)>=20]
  state11 -> state8 [order 3] : [abs(delta)>=10 && abs(delta)<15]{f20=0,f15=0,f10=0}
  state11 -> state1 [order 5] : [abs(delta)>=20]
  state1 -> state11 [order 3] : [abs(delta)>=2 && abs(delta)<5]
  data: delta input; sat output; kp output; f15 local; f20 local; f10 local; ki output; kd output; v local; reset output

== stateflow chart cpu1/Subsystem/Ready for deployment ==
  state state13
    sat = delta;
    kp= 0.35;
    if (abs(delta)<=0.5)
    ki=0.15;
    else
    ki=0.10;
    end
    reset = 1;
  state state12
    sat = delta;
    kp= 0.3;
    reset =0;
  state init
    f20 = 0;
    f15 = 0;
    f10 = 0;
    kp = 0;
    ki = 0;
    kd = 0;
    sat = 0;
  state else
    kp=0;
    sat=0;
    reset =1;
  state state10
    sat = delta;
    if f20 == 1 && f15==1 && f10==1
    kp = 0.07;
    elseif f20==0 && f15==1 && f10==1
    kp = 0.08;
    elseif f20==0 && f15==0 && f10==1
    kp = 0.08;
    else
    kp= 0.09;
    end
    reset =0;
  state state1
    if delta > 0
    sat = 20;
    else
    sat = -20;
    end
    kp = 0.025;
    f20 = 1;
    reset=0;
  state state9
    sat = delta ;
    if f20 == 1
    kp = 0.03;
    else
    kp = 0.04;
    end
    f15 = 1;
    reset=0;
  state state8
    sat = delta;
    if f20 == 1 && f15==1
    kp = 0.04;
    elseif f15==1 && f20==0
    kp = 0.045;
    else
    kp = 0.05;
    end
    f10 = 1;
    reset=0;
  state state11
    sat = delta;
    if f20 == 1 && f15==1 && f10==1
    kp = 0.15;
    elseif f20==0 && f15==1 && f10==1
    kp = 0.2;
    elseif f20==0 && f15==0 && f10==1
    kp = 0.2;
    else
    kp= 0.22;
    end
    reset =0;
  state13 -> state9 [order 5] : [abs(delta)<20 && abs(delta)>=15]{f20=0,f15=0,f10=0,ki=0}
  state13 -> state10 [order 3] : [abs(delta)>=5 && abs(delta)<10]{f20=0,f15=0,f10=0,ki=0}
  state13 -> state1 [order 6] : [abs(delta)>=20]{f20=0,f15=0,f10=0,ki=0}
  state13 -> state8 [order 4] : [abs(delta)>=10 && abs(delta)<15]{f20=0,f15=0,f10=0,ki=0}
  (junction 7) -> state13 [order 7] : [abs(delta)>=0.04 && abs(delta)<1]
  state8 -> state13 [order 7] : [abs(delta)>=0.04 && abs(delta)<1]
  state13 -> state12 [order 1] : [abs(delta)>=1 && abs(delta)<2]{f20=0,f15=0,f10=0,ki=0}
  state10 -> state13 [order 7] : [abs(delta)>=0.04 && abs(delta)<1]
  state13 -> else [order 7] : [abs(delta)<0.04]{ki=0}
  state9 -> state13 [order 7] : [abs(delta)>=0.04 && abs(delta)<1]
  (junction 7) -> state12 [order 6] : [abs(delta)>=1 && abs(delta)<2]
  state13 -> state11 [order 2] : [abs(delta)>=2 && abs(delta)<5]{f20=0,f15=0,f10=0,ki=0}
  state11 -> state13 [order 7] : [abs(delta)>=0.04 && abs(delta)<1]
  state12 -> state13 [order 7] : [abs(delta)>=0.04 && abs(delta)<1]
  state10 -> state1 [order 3] : [abs(delta)>=20]{f20=0,f15=0,f10=0}
  state12 -> state1 [order 5] : [abs(delta)>=20]
  (default) -> init
  state12 -> state10 [order 2] : [abs(delta)>=5 && abs(delta)<10]
  state1 -> state12 [order 6] : [abs(delta)>=1 && abs(delta)<2]
  state10 -> state12 [order 6] : [abs(delta)>=1 && abs(delta)<2]
  else -> (junction 7) : [~(abs(delta)<0.04)]{f20=0,f15=0,f10=0,reset=0}
  state12 -> else [order 6] : [abs(delta)<0.04]
  state9 -> state12 [order 6] : [abs(delta)>=1 && abs(delta)<2]
  state8 -> state12 [order 6] : [abs(delta)>=1 && abs(delta)<2]
  state1 -> state10 [order 3] : [abs(delta)>=5 && abs(delta)<10]{f20=0}
  state11 -> else [order 1] : [abs(delta)<0.04]
  state12 -> state9 [order 4] : [abs(delta)<20 && abs(delta)>=15]
  state12 -> state8 [order 3] : [abs(delta)>=10 && abs(delta)<15]
  state11 -> state12 [order 6] : [abs(delta)>=1 && abs(delta)<2]
  state12 -> state11 [order 1] : [abs(delta)>=2 && abs(delta)<5]
  state1 -> else [order 4] : [abs(delta)<0.04]
  state9 -> else [order 4] : [abs(delta)<0.04]
  state8 -> else [order 4] : [abs(delta)<0.04]
  state10 -> else [order 4] : [abs(delta)<0.04]
  init -> (junction 7)
  state11 -> state10 [order 2] : [abs(delta)>=5 && abs(delta)<10]{f20=0,f15=0,f10=0}
  state9 -> state10 [order 3] : [abs(delta)>=5 && abs(delta)<10]{f20=0,f15=0,f10=0}
  (junction 7) -> state1 [order 1] : [abs(delta)>=20]
  (junction 7) -> state10 [order 4] : [abs(delta)>=5 && abs(delta)<10]
  (junction 7) -> state11 [order 5] : [abs(delta)>=2 && abs(delta)<5]
  (junction 7) -> state8 [order 2] : [abs(delta)>=10 && abs(delta)<15]
  (junction 7) -> state9 [order 3] : [abs(delta)<20 && abs(delta)>=15]
  state10 -> state11 [order 5] : [abs(delta)>=2 && abs(delta)<5]
  state8 -> state1 [order 1] : [abs(delta)>=20]
  state10 -> state9 [order 2] : [abs(delta)<20 && abs(delta)>=15]{f20=0,f15=0,f10=0}
  state8 -> state10 [order 3] : [abs(delta)>=5 && abs(delta)<10]
  state10 -> state8 [order 1] : [abs(delta)>=10 && abs(delta)<15]{f20=0,f15=0,f10=0}
  state11 -> state1 [order 5] : [abs(delta)>=20]
  state9 -> state1 [order 2] : [abs(delta)>=20]
  state1 -> state9 [order 1] : [abs(delta)<20 && abs(delta)>=15]
  state1 -> state8 [order 2] : [abs(delta)>=10 && abs(delta)<15]{f20=0}
  state1 -> state11 [order 5] : [abs(delta)>=2 && abs(delta)<5]
  state8 -> state9 [order 2] : [abs(delta)<20 && abs(delta)>=15]{f20=0}
  state9 -> state8 [order 1] : [abs(delta)>=10 && abs(delta)<15]
  state11 -> state9 [order 4] : [abs(delta)<20 && abs(delta)>=15]{f20=0,f15=0,f10=0}
  state9 -> state11 [order 5] : [abs(delta)>=2 && abs(delta)<5]
  state8 -> state11 [order 5] : [abs(delta)>=2 && abs(delta)<5]
  state11 -> state8 [order 3] : [abs(delta)>=10 && abs(delta)<15]{f20=0,f15=0,f10=0}
  data: delta input; sat output single; kp output; f15 local; f20 local; f10 local; ki output; kd output; v local; reset output

== stateflow chart cpu1/Subsystem/Chart2 ==
  state state13
    sat = double(delta);
    kp= 0.35;
    if (abs(delta)<=0.5)
    ki=0.15;
    else
    ki=0.10;
    end
    reset = 1;
  state state12
    if delta > 0
    sat = 1;
    else
    sat = -1;
    end
    kp= 0.3;
    reset =0;
  state init
    f20 = 0;
    f15 = 0;
    f10 = 0;
    kp = 0;
    ki = 0;
    kd = 0;
    sat = 0;
  state else
    kp=0;
    sat=0;
    reset =1;
  state state10
    if delta > 0
    sat = 5;
    else
    sat = -5;
    end
    if f20 == 1 && f15==1 && f10==1
    kp = 0.07;
    elseif f20==0 && f15==1 && f10==1
    kp = 0.08;
    elseif f20==0 && f15==0 && f10==1
    kp = 0.08;
    else
    kp= 0.09;
    end
    reset =0;
  state state1
    if delta > 0
    sat = 20;
    else
    sat = -20;
    end
    kp = 0.03;
    f20 = 1;
    reset=0;
  state state9
    if delta > 0
    sat = 15;
    else
    sat = -15;
    end
    if f20 == 1
    kp = 0.03;
    else
    kp = 0.04;
    end
    f15 = 1;
    reset=0;
  state state8
    if delta > 0
    sat = 10;
    else
    sat = -10;
    end
    if f20 == 1 && f15==1
    kp = 0.04;
    elseif f15==1 && f20==0
    kp = 0.045;
    else
    kp = 0.05;
    end
    f10 = 1;
    reset=0;
  state state11
    if delta > 0
    sat = 2;
    else
    sat = -2;
    end
    if f20 == 1 && f15==1 && f10==1
    kp = 0.15;
    elseif f20==0 && f15==1 && f10==1
    kp = 0.2;
    elseif f20==0 && f15==0 && f10==1
    kp = 0.2;
    else
    kp= 0.22;
    end
    reset =0;
  state13 -> state9 [order 5] : [abs(delta)<20 && abs(delta)>=15]{f20=0,f15=0,f10=0,ki=0}
  state13 -> state10 [order 3] : [abs(delta)>=5 && abs(delta)<10]{f20=0,f15=0,f10=0,ki=0}
  state13 -> state1 [order 6] : [abs(delta)>=20]{f20=0,f15=0,f10=0,ki=0}
  state13 -> state8 [order 4] : [abs(delta)>=10 && abs(delta)<15]{f20=0,f15=0,f10=0,ki=0}
  (junction 7) -> state13 [order 7] : [abs(delta)>=0.04 && abs(delta)<1]
  state8 -> state13 [order 7] : [abs(delta)>=0.04 && abs(delta)<1]
  state13 -> state12 [order 1] : [abs(delta)>=1 && abs(delta)<2]{f20=0,f15=0,f10=0,ki=0}
  state10 -> state13 [order 7] : [abs(delta)>=0.04 && abs(delta)<1]
  state13 -> else [order 7] : [abs(delta)<0.04]{ki=0}
  state9 -> state13 [order 7] : [abs(delta)>=0.04 && abs(delta)<1]
  (junction 7) -> state12 [order 6] : [abs(delta)>=1 && abs(delta)<2]
  state13 -> state11 [order 2] : [abs(delta)>=2 && abs(delta)<5]{f20=0,f15=0,f10=0,ki=0}
  state11 -> state13 [order 7] : [abs(delta)>=0.04 && abs(delta)<1]
  state12 -> state13 [order 7] : [abs(delta)>=0.04 && abs(delta)<1]
  state10 -> state1 [order 3] : [abs(delta)>=20]{f20=0,f15=0,f10=0}
  state12 -> state1 [order 5] : [abs(delta)>=20]
  (default) -> init
  state12 -> state10 [order 2] : [abs(delta)>=5 && abs(delta)<10]
  state1 -> state12 [order 6] : [abs(delta)>=1 && abs(delta)<2]
  state10 -> state12 [order 6] : [abs(delta)>=1 && abs(delta)<2]
  else -> (junction 7) : [~(abs(delta)<0.04)]{f20=0,f15=0,f10=0,reset=0}
  state12 -> else [order 6] : [abs(delta)<0.04]
  state9 -> state12 [order 6] : [abs(delta)>=1 && abs(delta)<2]
  state8 -> state12 [order 6] : [abs(delta)>=1 && abs(delta)<2]
  state11 -> else [order 1] : [abs(delta)<0.04]
  state1 -> state10 [order 3] : [abs(delta)>=5 && abs(delta)<10]{f20=0}
  state12 -> state9 [order 4] : [abs(delta)<20 && abs(delta)>=15]
  state12 -> state8 [order 3] : [abs(delta)>=10 && abs(delta)<15]
  state11 -> state12 [order 6] : [abs(delta)>=1 && abs(delta)<2]
  state12 -> state11 [order 1] : [abs(delta)>=2 && abs(delta)<5]
  state1 -> else [order 4] : [abs(delta)<0.04]
  state9 -> else [order 4] : [abs(delta)<0.04]
  state8 -> else [order 4] : [abs(delta)<0.04]
  state10 -> else [order 4] : [abs(delta)<0.04]
  init -> (junction 7)
  state11 -> state10 [order 2] : [abs(delta)>=5 && abs(delta)<10]{f20=0,f15=0,f10=0}
  state9 -> state10 [order 3] : [abs(delta)>=5 && abs(delta)<10]{f20=0,f15=0,f10=0}
  (junction 7) -> state1 [order 1] : [abs(delta)>=20]
  (junction 7) -> state10 [order 4] : [abs(delta)>=5 && abs(delta)<10]
  (junction 7) -> state11 [order 5] : [abs(delta)>=2 && abs(delta)<5]
  (junction 7) -> state8 [order 2] : [abs(delta)>=10 && abs(delta)<15]
  (junction 7) -> state9 [order 3] : [abs(delta)<20 && abs(delta)>=15]
  state10 -> state11 [order 5] : [abs(delta)>=2 && abs(delta)<5]
  state8 -> state1 [order 1] : [abs(delta)>=20]
  state11 -> state1 [order 5] : [abs(delta)>=20]
  state10 -> state9 [order 2] : [abs(delta)<20 && abs(delta)>=15]{f20=0,f15=0,f10=0}
  state8 -> state10 [order 3] : [abs(delta)>=5 && abs(delta)<10]
  state10 -> state8 [order 1] : [abs(delta)>=10 && abs(delta)<15]{f20=0,f15=0,f10=0}
  state9 -> state1 [order 2] : [abs(delta)>=20]
  state1 -> state8 [order 2] : [abs(delta)>=10 && abs(delta)<15]{f20=0}
  state1 -> state9 [order 1] : [abs(delta)<20 && abs(delta)>=15]
  state1 -> state11 [order 5] : [abs(delta)>=2 && abs(delta)<5]
  state8 -> state9 [order 2] : [abs(delta)<20 && abs(delta)>=15]{f20=0}
  state9 -> state8 [order 1] : [abs(delta)>=10 && abs(delta)<15]
  state11 -> state9 [order 4] : [abs(delta)<20 && abs(delta)>=15]{f20=0,f15=0,f10=0}
  state9 -> state11 [order 5] : [abs(delta)>=2 && abs(delta)<5]
  state8 -> state11 [order 5] : [abs(delta)>=2 && abs(delta)<5]
  state11 -> state8 [order 3] : [abs(delta)>=10 && abs(delta)<15]{f20=0,f15=0,f10=0}
  data: delta input; sat output; kp output; f15 local; f20 local; f10 local; ki output; kd output; v local; reset output

== matlab function cpu1/Subsystem/5od balak haishift/1st region ==
  data: x input; y output
function y = map(x)
in_min = 0;
in_max = 511;
out_min = -179;
out_max = 180;

y = ((x - in_min) * (out_max - out_min)/ (in_max - in_min)) + out_min;

== matlab function cpu1/Subsystem1/map_angle1 ==
  data: enc_value input; range input; angle output
function angle = map_angle(enc_value, range)
    angle = enc_value;
    if range == -2
        angle = enc_value - 720;
    elseif range == -1
        angle = enc_value - 360;
    elseif range == 0
        angle = enc_value;
    elseif range == 1
        angle = enc_value + 360;
    elseif range == 2
        angle = enc_value + 720;
    end
end

== matlab function cpu1/Subsystem1/MATLAB Function1 ==
  data: u input; y output
function y = fcn(u)

u = transpose(u)
e = u(1,9)
i=8;
while i>0
 e = bitor(bitsll(e,1)  ,bitxor(u(1,i) , bitand(e ,1)))
 i=i-1
 end
y = e

== matlab function cpu1/Subsystem1/Mapping ==
  data: enc input; y_final output; pot input
function y_final = map(enc,pot)
in_min = 0;
in_max = 511;
out_min = -179;
out_max = 180;

y = (enc - in_min) * (out_max - out_min) / (in_max - in_min) + out_min;
if(pot < 695)
    in_min = 0;
    in_max = 511;
    out_min = -899;
    out_max = -540;
elseif ( bitand(pot >= 695, pot < 766) )
    if ( y >= 150 )
        in_min = 0;
        in_max = 511;
        out_min = -899;
        out_max = -540;
    elseif ( y <= -149 )
        in_min = 0;
        in_max = 511;
        out_min = -539;
        out_max = -180;
    end
elseif (bitand(pot >= 766 , pot < 1129) )
    in_min = 0;
    in_max = 511;
    out_min = -539;
    out_max = -180;
    
    % Region between First & Second Turns
elseif ( bitand(pot >= 1129 , pot < 1200) )
    if ( y >= 150 )
        in_min = 0;
        in_max = 511;
        out_min = -539;
        out_max = -180;
    elseif ( y <= -149 )
        in_min = 0;
        in_max = 511;
        out_min = -179;
        out_max = 180;
    end
    % Clockwise Mapping %
    
    % First Turn
    %if ( bitand(pot >= 409.3 , pot <511.99) )
elseif ( bitand(pot >= 1200 , pot < 1559) )
    in_min = 0;
    in_max = 511;
    out_min = -179;
    out_max = 180;
    
    % Region between First & Second Turns
elseif ( bitand(pot >= 1559  , pot < 1627) )
    if ( y >= 150 )
        in_min = 0;
        in_max = 511;
        out_min = -179;
        out_max = 180;
    elseif ( y <= -149 )
        in_min = 0;
        in_max = 511;
        out_min = 181;
        out_max = 540;
    end
    
elseif ( bitand(pot >= 1627 , pot < 1995) )
    in_min = 0;
    in_max = 511;
    out_min = 181;
    out_max = 540;
    
elseif ( bitand(pot >= 1995 , pot < 2071) )
    if (  y >= 150 )
        in_min = 0;
        in_max = 511;
        out_min = 181;
        out_max = 540;
    elseif ( y <= -149 )
        in_min = 0;
        in_max = 511;
        out_min = 541;
        out_max = 900;
    end
    
elseif (pot >= 2071)
    in_min = 0;
    in_max = 511;
    out_min = 541;
    out_max = 900;
    
end




y_final = (enc - in_min) * (out_max - out_min) / (in_max - in_min) + out_min;

== matlab function cpu1/Subsystem1/Steering Ratio (polo) ==
  data: u input; y output
function y = map(u)

%y = (-9.6071*x) + 38.714;

% y = (0.052739*x) - 1.7711;
% y = ((-4.988350733322303e-06)*(u^2)) + 0.0570*u + 0.3624;
y = ((-3.781939053610847e-06)*(u^2)) + 0.0579*u + 0.1094;

== matlab function cpu1/Subsystem/5od balak haishift/MATLAB Function1 ==
  data: u input; y output
function y = fcn(u)

u = transpose(u)
e = u(1,9)
i=8;
while i>0
 e = bitor(bitsll(e,1)  ,bitxor(u(1,i) , bitand(e ,1)))
 i=i-1
 end
y = e

== matlab function cpu1/Subsystem/5od balak haishift/MATLAB Function2 ==
  data: u input; y output; x input
function y = fcn(u,x)
if (u==0 && x ==511)
    z= 360/512;
elseif (u==511 && x==0)
    z=-360/512;
else 
    z= (u-x)*360/512;
end
y = z;

== matlab function cpu1/Subsystem/5od balak haishift/Mapping ==
  data: enc input; y_final output; pot input
function y_final = map(enc,pot)
in_min = 0;
in_max = 511;
out_min = -179;
out_max = 180;

y = (enc - in_min) * (out_max - out_min) / (in_max - in_min) + out_min;
if(pot < 695)
    in_min = 0;
    in_max = 511;
    out_min = -899;
    out_max = -540;
elseif ( bitand(pot >= 695, pot < 766) )
    if ( y >= 150 )
        in_min = 0;
        in_max = 511;
        out_min = -899;
        out_max = -540;
    elseif ( y <= -149 )
        in_min = 0;
        in_max = 511;
        out_min = -539;
        out_max = -180;
    end
elseif (bitand(pot >= 766 , pot < 1129) )
    in_min = 0;
    in_max = 511;
    out_min = -539;
    out_max = -180;
    
    % Region between First & Second Turns
elseif ( bitand(pot >= 1129 , pot < 1200) )
    if ( y >= 150 )
        in_min = 0;
        in_max = 511;
        out_min = -539;
        out_max = -180;
    elseif ( y <= -149 )
        in_min = 0;
        in_max = 511;
        out_min = -179;
        out_max = 180;
    end
    % Clockwise Mapping %
    
    % First Turn
    %if ( bitand(pot >= 409.3 , pot <511.99) )
elseif ( bitand(pot >= 1200 , pot < 1559) )
    in_min = 0;
    in_max = 511;
    out_min = -179;
    out_max = 180;
    
    % Region between First & Second Turns
elseif ( bitand(pot >= 1559  , pot < 1627) )
    if ( y >= 150 )
        in_min = 0;
        in_max = 511;
        out_min = -179;
        out_max = 180;
    elseif ( y <= -149 )
        in_min = 0;
        in_max = 511;
        out_min = 181;
        out_max = 540;
    end
    
elseif ( bitand(pot >= 1627 , pot < 1995) )
    in_min = 0;
    in_max = 511;
    out_min = 181;
    out_max = 540;
    
elseif ( bitand(pot >= 1995 , pot < 2071) )
    if (  y >= 150 )
        in_min = 0;
        in_max = 511;
        out_min = 181;
        out_max = 540;
    elseif ( y <= -149 )
        in_min = 0;
        in_max = 511;
        out_min = 541;
        out_max = 900;
    end
    
elseif (pot >= 2071)
    in_min = 0;
    in_max = 511;
    out_min = 541;
    out_max = 900;
    
end




y_final = (enc - in_min) * (out_max - out_min) / (in_max - in_min) + out_min;

== matlab function cpu1/Subsystem/5od balak haishift/Steering Ratio (polo) ==
  data: u input; y output
function y = map(u)

%y = (-9.6071*x) + 38.714;

% y = (0.052739*x) - 1.7711;
% y = ((-4.988350733322303e-06)*(u^2)) + 0.0570*u + 0.3624;
y = ((-3.781939053610847e-06)*(u^2)) + 0.0579*u + 0.1094;
